simulink model "rural_capacity_model"  (R2026a)
settings: Solver=VariableStepAuto  StopTime=30
libraries: simulink x2

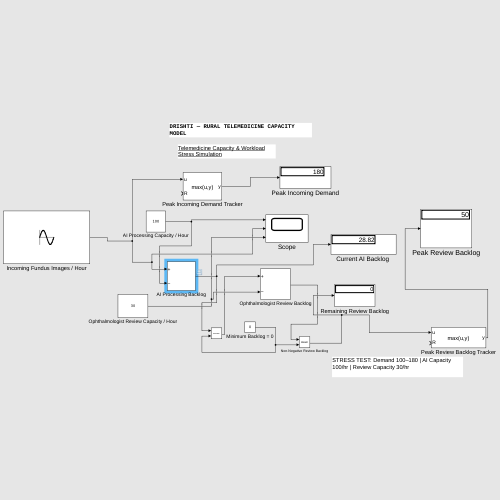
[thumbnail: Simulink's stored preview of the top-level diagram]
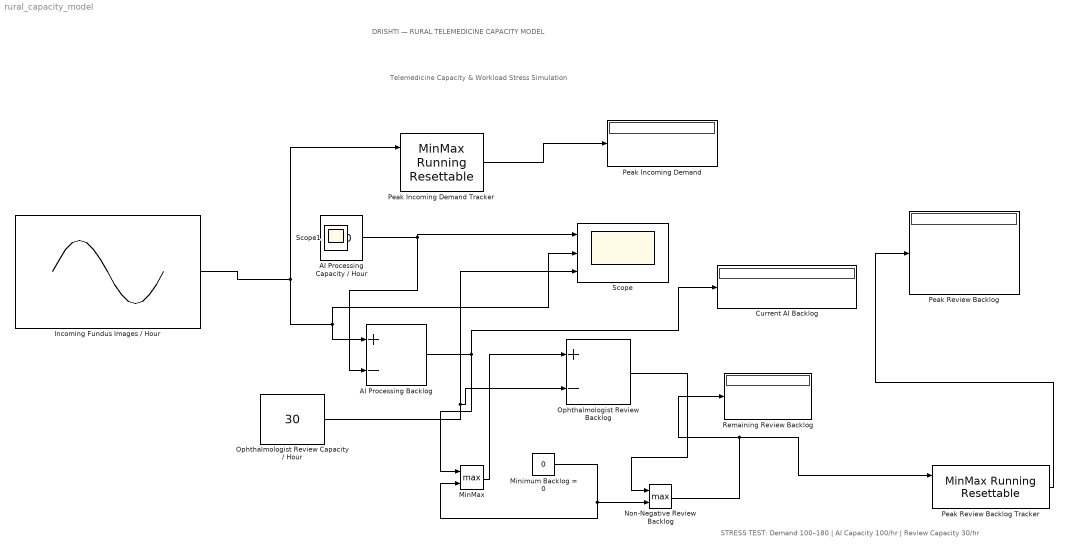
== system rural_capacity_model ==
  note: STRESS TEST: Demand 100–180 | AI Capacity 100/hr | Review Capacity 30/hr
  note: Telemedicine Capacity & Workload Stress Simulation
  note: DRISHTI — RURAL TELEMEDICINE CAPACITY MODEL
  AI Processing Backlog : Sum  Inputs=+-
  AI Processing Capacity / Hour : Constant  Value=100
  "Current AI Backlog " : Display
  Incoming Fundus Images / Hour : Sin  Amplitude=40  Bias=140  Frequency=0.2  SampleTime=0
  MinMax : MinMax  Function=max  Inputs=2
  Minimum Backlog = 0 : Constant  Value=0
  Non-Negative Review Backlog : MinMax  Function=max  Inputs=2
  Ophthalmologist Review Backlog : Sum  Inputs=+-
  Ophthalmologist Review Capacity / Hour : Constant  Value=30
  Peak Incoming Demand : Display
  Peak Incoming Demand Tracker : simulink/Math Operations/MinMax Running Resettable  Function=max  vinit=0.0
  Peak Review Backlog : Display
  Peak Review Backlog Tracker : simulink/Math Operations/MinMax Running Resettable  Function=max  vinit=0.0
  Remaining Review Backlog : Display
  Scope : Scope  NumInputPorts=3
      settings: TimeSpan=30  ActiveDisplayYMinimum=11.250291398850173  ActiveDisplayYMaximum=198.74737741034846
  Scope1 : Scope
      settings: ActiveDisplayYMinimum=-9.9996287444880654  ActiveDisplayYMaximum=89.997368537386066
  wires:
  AI Processing Capacity / Hour/1 -> AI Processing Backlog/2, Scope/1
  AI Processing Backlog/1 -> MinMax/1, "Current AI Backlog "/1
  Incoming Fundus Images / Hour/1 -> Scope/2, AI Processing Backlog/1, Peak Incoming Demand Tracker/1
  Ophthalmologist Review Capacity / Hour/1 -> Scope/3, Ophthalmologist Review Backlog/2
  Ophthalmologist Review Backlog/1 -> Non-Negative Review Backlog/1
  Minimum Backlog = 0/1 -> MinMax/2, Non-Negative Review Backlog/2
  Non-Negative Review Backlog/1 -> Peak Review Backlog Tracker/1, Remaining Review Backlog/1
  MinMax/1 -> Ophthalmologist Review Backlog/1
  Peak Review Backlog Tracker/1 -> Peak Review Backlog/1
  Peak Incoming Demand Tracker/1 -> Peak Incoming Demand/1
